simulink model "Schimmel_Evan_lab_5_model"  (R2020b)
settings: Solver=VariableStepAuto  StartTime=0.0  StopTime=10.0  RelTol=1e-3
values from neighbouring files (symbols this model uses):
  Jd = 0.0014151    [Schimmel_Evan_lab_5_script.m]
  R = 0.133    [Schimmel_Evan_lab_5_script.m]
undefined symbols (not defined in the file or in its folder): Md
settings Model: Creator=schimmer  LastModifiedBy=schimmer

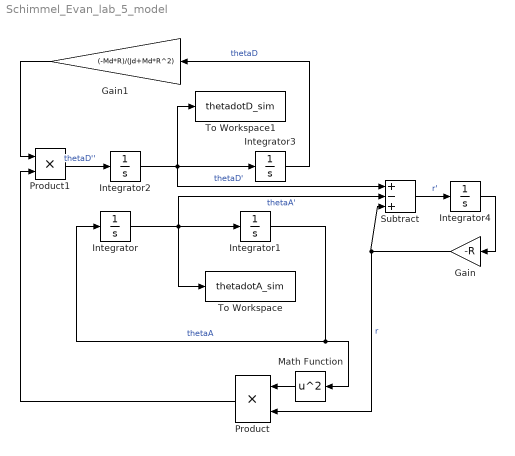
== system Schimmel_Evan_lab_5_model ==
  Gain : Gain  Gain=-R
  Gain1 : Gain  Gain=(-Md*R)/(Jd+Md*R^2)
  Integrator{,1..4} (5 alike) : Integrator
  Math Function : Math  Operator=square  SaturateOnIntegerOverflow=on
  Product : Product
  Product1 : Product
  Subtract : Sum  Inputs=+-+
  To Workspace : ToWorkspace  VariableName=thetadotA_sim  SaveFormat=Timeseries  SampleTime=-1
  To Workspace1 : ToWorkspace  VariableName=thetadotD_sim  SaveFormat=Timeseries  SampleTime=-1
  wires:
  Subtract/1 -> Integrator4/1  "r'"
  Integrator4/1 -> Gain/1
  Integrator2/1 -> Subtract/1, To Workspace1/1, Integrator3/1  "thetaD'"
  Integrator/1 -> Subtract/2, To Workspace/1, Integrator1/1  "thetaA'"
  Gain/1 -> Product/2, Subtract/3  "r"
  Integrator3/1 -> Gain1/1  "thetaD"
  Integrator1/1 -> Math Function/1, Integrator/1  "thetaA"
  Gain1/1 -> Product1/1
  Math Function/1 -> Product/1
  Product/1 -> Product1/2
  Product1/1 -> Integrator2/1  "thetaD''"
